simulink model "inverted_pendulum_on_cart3d"  (R2019a)
settings: Solver=VariableStepAuto  StartTime=0.0  StopTime=30  RelTol=1e-3
values from neighbouring files (symbols this model uses):
  b = 0.1    [Inverted_pendulum_on_cart.mat]
  g = 9.8    [Inverted_pendulum_on_cart.mat]
  I = 0.006    [Inverted_pendulum_on_cart.mat]
  l = 0.3    [Inverted_pendulum_on_cart.mat]
  M = 0.5    [Inverted_pendulum_on_cart.mat]
  m = 0.2    [Inverted_pendulum_on_cart.mat]
libraries: simulink x2
settings Model: Creator=Ranish  LastModifiedBy=Ranish

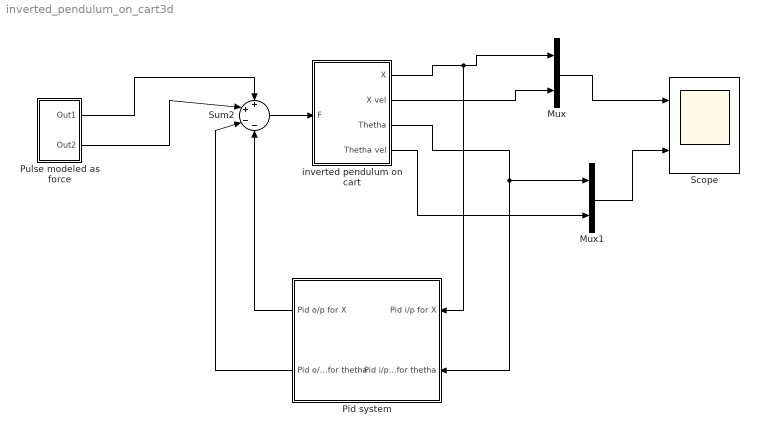
== system inverted_pendulum_on_cart3d ==
  Mux : Mux  Inputs=2
  Mux1 : Mux  Inputs=2
  Pid system : Subsystem
  "Pulse modeled as force " : Subsystem
  Scope : Scope  NumInputPorts=2
  Sum2 : Sum  Inputs=++--
  "inverted pendulum on cart " : Subsystem
  wires:
  Sum2/1 -> "inverted pendulum on cart "/1(F)
  "inverted pendulum on cart "/1("X ") -> Pid system/1(Pid i/p for X), Mux/1
  Mux/1 -> Scope/1
  "inverted pendulum on cart "/4("Thetha vel ") -> Mux1/2
  Mux1/1 -> Scope/2
  "inverted pendulum on cart "/3("Thetha ") -> Pid system/2(Pid i/p for thetha), Mux1/1
  "inverted pendulum on cart "/2("X vel ") -> Mux/2
  "Pulse modeled as force "/1(Out1) -> Sum2/1
  "Pulse modeled as force "/2(Out2) -> Sum2/2
  Pid system/2(Pid o/p for thetha) -> Sum2/3
  Pid system/1(Pid o/p for X) -> Sum2/4

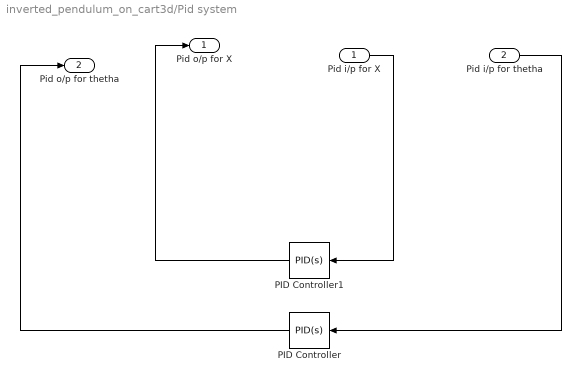
== system inverted_pendulum_on_cart3d/Pid system ==
  Pid i/p for X : Inport
  Pid i/p for thetha : Inport  Port=2
  PID Controller : simulink/Continuous/PID Controller  Controller=PID  Form=Parallel  TimeDomain=Continuous-time  SampleTime=-1  IntegratorMethod=Forward Euler  FilterMethod=Forward Euler  ControllerParametersSource=internal  P=1054.16123700867  I=2212.68658629558  D=61.4720921565294  UseFilter=on  N=31981.1269322279  TunerSelectOption=Transfer Function Based (PID Tuner App)  InitialConditionSource=internal  InitialConditionForIntegrator=0  InitialConditionForFilter=0  DifferentiatorICPrevScaledInput=0  ExternalReset=none  TrackingMode=off  Kt=1  LimitOutput=off  UpperSaturationLimit=inf  LowerSaturationLimit=-inf  LinearizeAsGain=on  AntiWindupMode=none  Kb=1  POutMin=[]  POutMax=[]  IOutMin=[]  IOutMax=[]  DOutMin=[]  DOutMax=[]  NOutMin=[]  NOutMax=[]  SumOutMin=[]  SumOutMax=[]  SaturationOutMin=[]  SaturationOutMax=[]  PParamMin=[]  PParamMax=[]  IParamMin=[]  IParamMax=[]  DParamMin=[]  DParamMax=[]  NParamMin=[]  NParamMax=[]  KbParamMin=[]  KbParamMax=[]  KtParamMin=[]  KtParamMax=[]  KbOutMin=[]  KbOutMax=[]  KtOutMin=[]  KtOutMax=[]  IntegratorOutMin=[]  IntegratorOutMax=[]  FilterOutMin=[]  FilterOutMax=[]  SumI1OutMin=[]  SumI1OutMax=[]  SumI2OutMin=[]  SumI2OutMax=[]  SumI3OutMin=[]  SumI3OutMax=[]  SumI4OutMin=[]  SumI4OutMax=[]  SumDOutMin=[]  SumDOutMax=[]  DifferentiatorOutMin=[]  DifferentiatorOutMax=[]  FilterDiffOutCoefMin=[]  FilterDiffOutCoefMax=[]  ReciprocalOutMin=[]  ReciprocalOutMax=[]  SumDenOutMin=[]  SumDenOutMax=[]  SumNumOutMin=[]  SumNumOutMax=[]  DivideOutMin=[]  DivideOutMax=[]  IntegratorContinuousStateAttributes=''  IntegratorStateMustResolveToSignalObject=off  IntegratorRTWStateStorageClass=Auto  FilterContinuousStateAttributes=''  FilterStateMustResolveToSignalObject=off  FilterRTWStateStorageClass=Auto  ParallelPVariant=InternalParameters  IdealPVariant=Disabled  IVariant=InternalParameters  DVariant=InternalParameters  IntegratorVariant=Continuous  SatVariant=Disabled  AWVariant=Passthrough  PCopyVariant=Disabled  TRVariant=Disabled  FdbkBlocksVariant=Forward  IdealPFdbkVariant=Disabled  SatFdbkVariant=Disabled  DerivativeFilterVariant=ContFilter  NVariant=InternalParameters  NCopyVariant=Disabled  FilterICVariant=InternalICsFilter  IntegratorICVariant=InternalICs  ExternalResetVariant=Disabled  TRSumVariant=Passthrough  SumFdbkVariant=Disabled  SumVariant=Sum_PID
  PID Controller1 : simulink/Continuous/PID Controller  Controller=PID  Form=Parallel  TimeDomain=Continuous-time  SampleTime=-1  IntegratorMethod=Forward Euler  FilterMethod=Forward Euler  ControllerParametersSource=internal  P=-355.812530075887  I=-50.0553195874022  D=2.1115923912323  UseFilter=on  N=168.504362656961  TunerSelectOption=Transfer Function Based (PID Tuner App)  InitialConditionSource=internal  InitialConditionForIntegrator=0  InitialConditionForFilter=0  DifferentiatorICPrevScaledInput=0  ExternalReset=none  TrackingMode=off  Kt=1  LimitOutput=off  UpperSaturationLimit=inf  LowerSaturationLimit=-inf  LinearizeAsGain=on  AntiWindupMode=none  Kb=1  POutMin=[]  POutMax=[]  IOutMin=[]  IOutMax=[]  DOutMin=[]  DOutMax=[]  NOutMin=[]  NOutMax=[]  SumOutMin=[]  SumOutMax=[]  SaturationOutMin=[]  SaturationOutMax=[]  PParamMin=[]  PParamMax=[]  IParamMin=[]  IParamMax=[]  DParamMin=[]  DParamMax=[]  NParamMin=[]  NParamMax=[]  KbParamMin=[]  KbParamMax=[]  KtParamMin=[]  KtParamMax=[]  KbOutMin=[]  KbOutMax=[]  KtOutMin=[]  KtOutMax=[]  IntegratorOutMin=[]  IntegratorOutMax=[]  FilterOutMin=[]  FilterOutMax=[]  SumI1OutMin=[]  SumI1OutMax=[]  SumI2OutMin=[]  SumI2OutMax=[]  SumI3OutMin=[]  SumI3OutMax=[]  SumI4OutMin=[]  SumI4OutMax=[]  SumDOutMin=[]  SumDOutMax=[]  DifferentiatorOutMin=[]  DifferentiatorOutMax=[]  FilterDiffOutCoefMin=[]  FilterDiffOutCoefMax=[]  ReciprocalOutMin=[]  ReciprocalOutMax=[]  SumDenOutMin=[]  SumDenOutMax=[]  SumNumOutMin=[]  SumNumOutMax=[]  DivideOutMin=[]  DivideOutMax=[]  IntegratorContinuousStateAttributes=''  IntegratorStateMustResolveToSignalObject=off  IntegratorRTWStateStorageClass=Auto  FilterContinuousStateAttributes=''  FilterStateMustResolveToSignalObject=off  FilterRTWStateStorageClass=Auto  ParallelPVariant=InternalParameters  IdealPVariant=Disabled  IVariant=InternalParameters  DVariant=InternalParameters  IntegratorVariant=Continuous  SatVariant=Disabled  AWVariant=Passthrough  PCopyVariant=Disabled  TRVariant=Disabled  FdbkBlocksVariant=Forward  IdealPFdbkVariant=Disabled  SatFdbkVariant=Disabled  DerivativeFilterVariant=ContFilter  NVariant=InternalParameters  NCopyVariant=Disabled  FilterICVariant=InternalICsFilter  IntegratorICVariant=InternalICs  ExternalResetVariant=Disabled  TRSumVariant=Passthrough  SumFdbkVariant=Disabled  SumVariant=Sum_PID
  Pid o/p for X : Outport
  Pid o/p for thetha : Outport  Port=2
  wires:
  Pid i/p for thetha/1 -> PID Controller/1
  Pid i/p for X/1 -> PID Controller1/1
  PID Controller1/1 -> Pid o/p for X/1
  PID Controller/1 -> Pid o/p for thetha/1

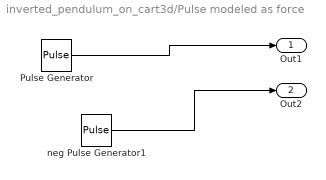
== system inverted_pendulum_on_cart3d/Pulse modeled as force  ==
  Pulse Generator : DiscretePulseGenerator  PulseType=Time based  Amplitude=1000  Period=30  PulseWidth=5
  neg Pulse Generator1 : DiscretePulseGenerator  PulseType=Time based  Amplitude=-1000  Period=30  PulseWidth=5  PhaseDelay=15
  Out1 : Outport
  Out2 : Outport  Port=2
  wires:
  Pulse Generator/1 -> Out1/1
  neg Pulse Generator1/1 -> Out2/1

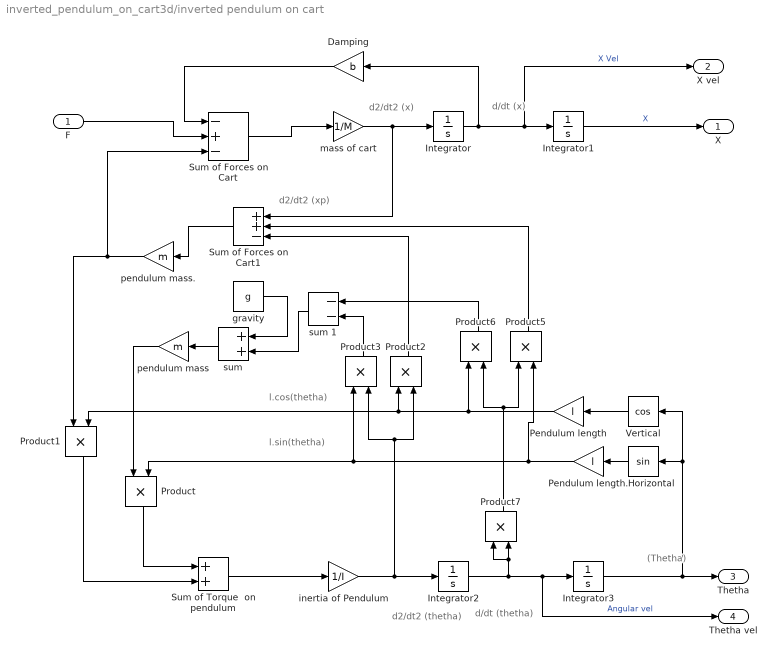
== system inverted_pendulum_on_cart3d/inverted pendulum on cart  ==
  note: l.cos(thetha)
  note: (Thetha)
  note: d/dt (thetha)
  note: d2/dt2 (thetha)
  note: d/dt (x)
  note: d2/dt2 (x)
  note: d2/dt2 (xp)
  note: l.sin(thetha)
  F : Inport
  Damping : Gain  Gain=b
  Horizontal : Trigonometry
  Integrator{,1..3} (4 alike) : Integrator
  Pendulum length : Gain  Gain=l
  Pendulum length. : Gain  Gain=l
  Product{,1..3,5..7} (7 alike) : Product
  Sum of Forces on Cart : Sum  Inputs=-+-
  Sum of Forces on Cart1 : Sum  Inputs=++-
  Sum of Torque  on pendulum : Sum
  Vertical : Trigonometry  Operator=cos
  gravity : Constant  Value=g
  "inertia of Pendulum " : Gain  Gain=1/I
  mass of cart : Gain  Gain=1/M
  "pendulum mass " : Gain  Gain=m
  "pendulum mass. " : Gain  Gain=m
  "sum " : Sum
  sum 1 : Sum  Inputs=--
  "X " : Outport
  "X vel " : Outport  Port=2
  "Thetha " : Outport  Port=3
  "Thetha vel " : Outport  Port=4
  wires:
  Integrator2/1 -> Integrator3/1, "Thetha vel "/1, Product7/1, Product7/2  "Angular vel"
  Integrator/1 -> Damping/1, "X vel "/1, Integrator1/1  "X Vel"
  Vertical/1 -> Pendulum length/1
  "inertia of Pendulum "/1 -> Integrator2/1, Product3/2, Product2/2
  Product5/1 -> Sum of Forces on Cart1/2
  Pendulum length./1 -> Product3/1, Product/2, Product5/2
  Sum of Torque  on pendulum/1 -> "inertia of Pendulum "/1
  mass of cart/1 -> Sum of Forces on Cart1/1, Integrator/1
  Product7/1 -> Product5/1, Product6/2
  Integrator3/1 -> "Thetha "/1, Horizontal/1, Vertical/1
  F/1 -> Sum of Forces on Cart/2
  Horizontal/1 -> Pendulum length./1
  "pendulum mass. "/1 -> Sum of Forces on Cart/3, Product1/1
  Integrator1/1 -> "X "/1  "X"
  Product/1 -> Sum of Torque  on pendulum/1
  Pendulum length/1 -> Product2/1, Product1/2, Product6/1
  gravity/1 -> "sum "/1
  Damping/1 -> Sum of Forces on Cart/1
  Sum of Forces on Cart/1 -> mass of cart/1
  Sum of Forces on Cart1/1 -> "pendulum mass. "/1
  "pendulum mass "/1 -> Product/1
  Product6/1 -> sum 1/1
  sum 1/1 -> "sum "/2
  Product2/1 -> Sum of Forces on Cart1/3
  "sum "/1 -> "pendulum mass "/1
  Product1/1 -> Sum of Torque  on pendulum/2
  Product3/1 -> sum 1/2
